simulink library "calcAttchPtStates_ul"  (R2018b)
settings: Solver=VariableStepAuto  StartTime=0.0  StopTime=10.0  RelTol=1e-3
values from neighbouring files (symbols this model uses):
  some_class = reshape(some_class,1,[])    [calcAttchPtStates_ts.m]
libraries: vrlib x1, eulAng2RotMat_ul x1
settings Model: Creator=Ayaz  LastModifiedBy=asiddiq2

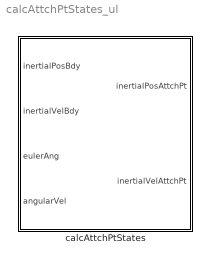
== system calcAttchPtStates_ul ==
  calcAttchPtStates : Subsystem  TreatAsAtomicUnit=on  mask{attchPt=some_class}
      mask prompts: attchPt "Tether attachment position vector"
      mask DialogControl ParameterGroupVar Prompt: Locations

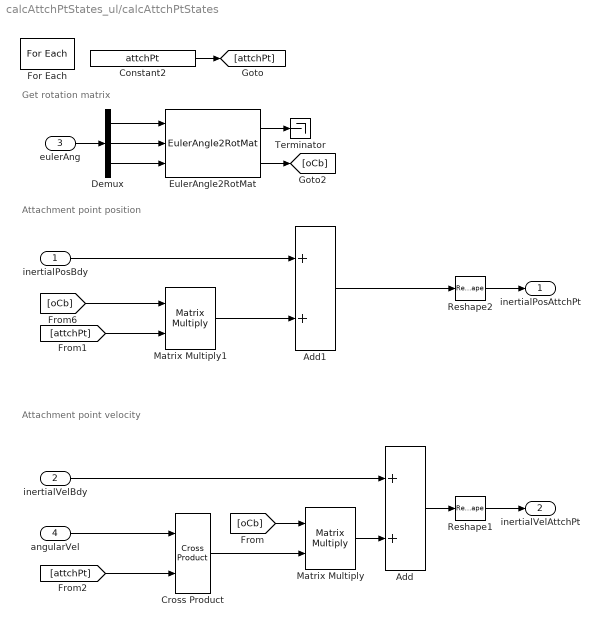
== system calcAttchPtStates_ul/calcAttchPtStates ==
  note: Get rotation matrix
  note: Attachment point position
  note: Attachment point velocity
  inertialPosBdy : Inport  PortDimensions=[3,1]
  inertialVelBdy : Inport  Port=2  PortDimensions=[3,1]
  eulerAng : Inport  Port=3  PortDimensions=[3,1]
  angularVel : Inport  Port=4  PortDimensions=[3,1]
  Add : Sum
  Add1 : Sum
  Constant2 : Constant  Value=attchPt  VectorParams1D=off
  Cross Product : vrlib/Utilities/Cross Product
      settings: SourceProductBaseCode=VR
  Demux : Demux  Outputs=3
  EulerAngle2RotMat : eulAng2RotMat_ul/EulerAngle2RotMat  SystemSampleTime=-1
  For Each : ForEach  DisableCoverage=on  IterateSubsysMaskParameter=on  SubsysMaskParameterIterationDimension=2  IndexMode=One-based
  Matrix Multiply : Product  Multiplication=Matrix(*)
  Matrix Multiply1 : Product  Multiplication=Matrix(*)
  Reshape1 : Reshape  OutputDimensionality=Column vector (2-D)
  Reshape2 : Reshape  OutputDimensionality=Column vector (2-D)
  Terminator : Terminator
  inertialPosAttchPt : Outport  PortDimensions=[3,1]  ConcatenationDimension=2
  inertialVelAttchPt : Outport  Port=2  PortDimensions=[3,1]  ConcatenationDimension=2
  wires:
  EulerAngle2RotMat/2 -> [oCb]
  Demux/3 -> EulerAngle2RotMat/3
  Demux/2 -> EulerAngle2RotMat/2
  Demux/1 -> EulerAngle2RotMat/1
  EulerAngle2RotMat/1 -> Terminator/1
  eulerAng/1 -> Demux/1
  [oCb] -> Matrix Multiply/1
  Add1/1 -> Reshape2/1
  inertialVelBdy/1 -> Add/1
  angularVel/1 -> Cross Product/1
  inertialPosBdy/1 -> Add1/1
  Matrix Multiply/1 -> Add/2
  [oCb] -> Matrix Multiply1/1
  [attchPt] -> Cross Product/2
  Matrix Multiply1/1 -> Add1/2
  Cross Product/1 -> Matrix Multiply/2
  [attchPt] -> Matrix Multiply1/2
  Add/1 -> Reshape1/1
  Reshape1/1 -> inertialVelAttchPt/1
  Reshape2/1 -> inertialPosAttchPt/1
  Constant2/1 -> [attchPt]
